simulink model "PD_LargeTimeCons"  (R2020b)
(part 4 of 4)

    td2*(td1*(0.00084023437500000005238864897449957*cos(t1)*cos(t5)*sin(t1) + 0.00042011718750000002619432448724979*cos(t1)^2*cos(t2)*cos(t3)*cos(t4)*sin(t5) - 0.00042011718750000002619432448724979*cos(t2)*cos(t3)*cos(t4)*sin(t1)^2*sin(t5) - 0.00042011718750000002619432448724979*cos(t1)^2*cos(t2)*sin(t3)*sin(t4)*sin(t5) - 0.00042011718750000002619432448724979*cos(t1)^2*cos(t3)*sin(t2)*sin(t4)*sin(t5) - 0.00042011718750000002619432448724979*cos(t1)^2*cos(t4)*sin(t2)*sin(t3)*sin(t5) + 0.00042011718750000002619432448724979*cos(t2)*sin(t1)^2*sin(t3)*sin(t4)*sin(t5) + 0.00042011718750000002619432448724979*cos(t3)*sin(t1)^2*sin(t2)*sin(t4)*sin(t5) + 0.00042011718750000002619432448724979*cos(t4)*sin(t1)^2*sin(t2)*sin(t3)*sin(t5)) + td6*(0.5*(0.00084023437500000005238864897449957*cos(t1)*cos(t2)*cos(t3)*sin(t4)*sin(t5) + 0.00084023437500000005238864897449957*cos(t1)*cos(t2)*cos(t4)*sin(t3)*sin(t5) + 0.00084023437500000005238864897449957*cos(t1)*cos(t3)*cos(t4)*sin(t2)*sin(t5) - 0.00084023437500000005238864897449957*cos(t1)*sin(t2)*sin(t3)*sin(t4)*sin(t5))*(cos(t1)*cos(t2)*sin(t3)*sin(t4)*sin(t5) - 1.0*cos(t1)*cos(t2)*cos(t3)*cos(t4)*sin(t5) - 1.0*cos(t5)*sin(t1) + cos(t1)*cos(t3)*sin(t2)*sin(t4)*sin(t5) + cos(t1)*cos(t4)*sin(t2)*sin(t3)*sin(t5)) + 0.5*(cos(t1)*cos(t2)*cos(t3)*sin(t4)*sin(t5) + cos(t1)*cos(t2)*cos(t4)*sin(t3)*sin(t5) + cos(t1)*cos(t3)*cos(t4)*sin(t2)*sin(t5) - 1.0*cos(t1)*sin(t2)*sin(t3)*sin(t4)*sin(t5))*(0.00084023437500000005238864897449957*cos(t1)*cos(t2)*sin(t3)*sin(t4)*sin(t5) - 0.00084023437500000005238864897449957*cos(t1)*cos(t2)*cos(t3)*cos(t4)*sin(t5) - 0.00084023437500000005238864897449957*cos(t5)*sin(t1) + 0.00084023437500000005238864897449957*cos(t1)*cos(t3)*sin(t2)*sin(t4)*sin(t5) + 0.00084023437500000005238864897449957*cos(t1)*cos(t4)*sin(t2)*sin(t3)*sin(t5)) + 0.5*(0.0016804687500000001047772979489991*cos(t2)*cos(t3)*sin(t1)*sin(t4)*sin(t5) + 0.0016804687500000001047772979489991*cos(t2)*cos(t4)*sin(t1)*sin(t3)*sin(t5) + 0.0016804687500000001047772979489991*cos(t3)*cos(t4)*sin(t1)*sin(t2)*sin(t5) - 0.0016804687500000001047772979489991*sin(t1)*sin(t2)*sin(t3)*sin(t4)*sin(t5))*(cos(t1)*cos(t5) - 1.0*cos(t2)*cos(t3)*cos(t4)*sin(t1)*sin(t5) + cos(t2)*sin(t1)*sin(t3)*sin(t4)*sin(t5) + cos(t3)*sin(t1)*sin(t2)*sin(t4)*sin(t5) + cos(t4)*sin(t1)*sin(t2)*sin(t3)*sin(t5)) + 0.5*(cos(t2)*cos(t3)*sin(t1)*sin(t4)*sin(t5) + cos(t2)*cos(t4)*sin(t1)*sin(t3)*sin(t5) + cos(t3)*cos(t4)*sin(t1)*sin(t2)*sin(t5) - 1.0*sin(t1)*sin(t2)*sin(t3)*sin(t4)*sin(t5))*(0.0016804687500000001047772979489991*cos(t1)*cos(t5) - 0.0016804687500000001047772979489991*cos(t2)*cos(t3)*cos(t4)*sin(t1)*sin(t5) + 0.0016804687500000001047772979489991*cos(t2)*sin(t1)*sin(t3)*sin(t4)*sin(t5) + 0.0016804687500000001047772979489991*cos(t3)*sin(t1)*sin(t2)*sin(t4)*sin(t5) + 0.0016804687500000001047772979489991*cos(t4)*sin(t1)*sin(t2)*sin(t3)*sin(t5))) - 1.0*td5*(0.00063017578125000003929148673087468*cos(2.0*t2)*cos(2.0*t3)*cos(2.0*t4)*sin(t5) - 0.00042011718750000002619432448724979*cos(t1)^2*sin(t5) - 0.00042011718750000002619432448724979*sin(t5) - 0.00063017578125000003929148673087468*cos(2.0*t2)*sin(2.0*t3)*sin(2.0*t4)*sin(t5) - 0.00063017578125000003929148673087468*cos(2.0*t3)*sin(2.0*t2)*sin(2.0*t4)*sin(t5) - 0.00063017578125000003929148673087468*cos(2.0*t4)*sin(2.0*t2)*sin(2.0*t3)*sin(t5) - 0.00021005859375000001309716224362489*cos(2.0*t1)*cos(2.0*t2)*cos(2.0*t3)*cos(2.0*t4)*sin(t5) + 0.00021005859375000001309716224362489*cos(2.0*t1)*cos(2.0*t2)*sin(2.0*t3)*sin(2.0*t4)*sin(t5) + 0.00021005859375000001309716224362489*cos(2.0*t1)*cos(2.0*t3)*sin(2.0*t2)*sin(2.0*t4)*sin(t5) + 0.00021005859375000001309716224362489*cos(2.0*t1)*cos(2.0*t4)*sin(2.0*t2)*sin(2.0*t3)*sin(t5) - 0.00021005859375000001309716224362489*sin(2.0*t1)*cos(t2)*cos(t3)*cos(t4)*cos(t5) + 0.00021005859375000001309716224362489*sin(2.0*t1)*cos(t2)*cos(t5)*sin(t3)*sin(t4) + 0.00021005859375000001309716224362489*sin(2.0*t1)*cos(t3)*cos(t5)*sin(t2)*sin(t4) + 0.00021005859375000001309716224362489*sin(2.0*t1)*cos(t4)*cos(t5)*sin(t2)*sin(t3) - 0.00042011718750000002619432448724979*cos(t1)*cos(t2)*cos(t3)*cos(t4)*cos(t5)*sin(t1) + 0.00042011718750000002619432448724979*cos(t1)*cos(t2)*cos(t5)*sin(t1)*sin(t3)*sin(t4) + 0.00042011718750000002619432448724979*cos(t1)*cos(t3)*cos(t5)*sin(t1)*sin(t2)*sin(t4) + 0.00042011718750000002619432448724979*cos(t1)*cos(t4)*cos(t5)*sin(t1)*sin(t2)*sin(t3))) + td3*(td1*(0.00084023437500000005238864897449957*cos(t1)*cos(t5)*sin(t1) + 0.00042011718750000002619432448724979*cos(t1)^2*cos(t2)*cos(t3)*cos(t4)*sin(t5) - 0.00042011718750000002619432448724979*cos(t2)*cos(t3)*cos(t4)*sin(t1)^2*sin(t5) - 0.00042011718750000002619432448724979*cos(t1)^2*cos(t2)*sin(t3)*sin(t4)*sin(t5) - 0.00042011718750000002619432448724979*cos(t1)^2*cos(t3)*sin(t2)*sin(t4)*sin(t5) - 0.00042011718750000002619432448724979*cos(t1)^2*cos(t4)*sin(t2)*sin(t3)*sin(t5) + 0.00042011718750000002619432448724979*cos(t2)*sin(t1)^2*sin(t3)*sin(t4)*sin(t5) + 0.00042011718750000002619432448724979*cos(t3)*sin(t1)^2*sin(t2)*sin(t4)*sin(t5) + 0.00042011718750000002619432448724979*cos(t4)*sin(t1)^2*sin(t2)*sin(t3)*sin(t5)) + td6*(0.5*(0.00084023437500000005238864897449957*cos(t1)*cos(t2)*cos(t3)*sin(t4)*sin(t5) + 0.00084023437500000005238864897449957*cos(t1)*cos(t2)*cos(t4)*sin(t3)*sin(t5) + 0.00084023437500000005238864897449957*cos(t1)*cos(t3)*cos(t4)*sin(t2)*sin(t5) - 0.00084023437500000005238864897449957*cos(t1)*sin(t2)*sin(t3)*sin(t4)*sin(t5))*(cos(t1)*cos(t2)*sin(t3)*sin(t4)*sin(t5) - 1.0*cos(t1)*cos(t2)*cos(t3)*cos(t4)*sin(t5) - 1.0*cos(t5)*sin(t1) + cos(t1)*cos(t3)*sin(t2)*sin(t4)*sin(t5) + cos(t1)*cos(t4)*sin(t2)*sin(t3)*sin(t5)) + 0.5*(cos(t1)*cos(t2)*cos(t3)*sin(t4)*sin(t5) + cos(t1)*cos(t2)*cos(t4)*sin(t3)*sin(t5) + cos(t1)*cos(t3)*cos(t4)*sin(t2)*sin(t5) - 1.0*cos(t1)*sin(t2)*sin(t3)*sin(t4)*sin(t5))*(0.00084023437500000005238864897449957*cos(t1)*cos(t2)*sin(t3)*sin(t4)*sin(t5) - 0.00084023437500000005238864897449957*cos(t1)*cos(t2)*cos(t3)*cos(t4)*sin(t5) - 0.00084023437500000005238864897449957*cos(t5)*sin(t1) + 0.00084023437500000005238864897449957*cos(t1)*cos(t3)*sin(t2)*sin(t4)*sin(t5) + 0.00084023437500000005238864897449957*cos(t1)*cos(t4)*sin(t2)*sin(t3)*sin(t5)) + 0.5*(0.0016804687500000001047772979489991*cos(t2)*cos(t3)*sin(t1)*sin(t4)*sin(t5) + 0.0016804687500000001047772979489991*cos(t2)*cos(t4)*sin(t1)*sin(t3)*sin(t5) + 0.0016804687500000001047772979489991*cos(t3)*cos(t4)*sin(t1)*sin(t2)*sin(t5) - 0.0016804687500000001047772979489991*sin(t1)*sin(t2)*sin(t3)*sin(t4)*sin(t5))*(cos(t1)*cos(t5) - 1.0*cos(t2)*cos(t3)*cos(t4)*sin(t1)*sin(t5) + cos(t2)*sin(t1)*sin(t3)*sin(t4)*sin(t5) + cos(t3)*sin(t1)*sin(t2)*sin(t4)*sin(t5) + cos(t4)*sin(t1)*sin(t2)*sin(t3)*sin(t5)) + 0.5*(cos(t2)*cos(t3)*sin(t1)*sin(t4)*sin(t5) + cos(t2)*cos(t4)*sin(t1)*sin(t3)*sin(t5) + cos(t3)*cos(t4)*sin(t1)*sin(t2)*sin(t5) - 1.0*sin(t1)*sin(t2)*sin(t3)*sin(t4)*sin(t5))*(0.0016804687500000001047772979489991*cos(t1)*cos(t5) - 0.0016804687500000001047772979489991*cos(t2)*cos(t3)*cos(t4)*sin(t1)*sin(t5) + 0.0016804687500000001047772979489991*cos(t2)*sin(t1)*sin(t3)*sin(t4)*sin(t5) + 0.0016804687500000001047772979489991*cos(t3)*sin(t1)*sin(t2)*sin(t4)*sin(t5) + 0.0016804687500000001047772979489991*cos(t4)*sin(t1)*sin(t2)*sin(t3)*sin(t5))) - 1.0*td5*(0.00063017578125000003929148673087468*cos(2.0*t2)*cos(2.0*t3)*cos(2.0*t4)*sin(t5) - 0.00042011718750000002619432448724979*cos(t1)^2*sin(t5) - 0.00042011718750000002619432448724979*sin(t5) - 0.00063017578125000003929148673087468*cos(2.0*t2)*sin(2.0*t3)*sin(2.0*t4)*sin(t5) - 0.00063017578125000003929148673087468*cos(2.0*t3)*sin(2.0*t2)*sin(2.0*t4)*sin(t5) - 0.00063017578125000003929148673087468*cos(2.0*t4)*sin(2.0*t2)*sin(2.0*t3)*sin(t5) - 0.00021005859375000001309716224362489*cos(2.0*t1)*cos(2.0*t2)*cos(2.0*t3)*cos(2.0*t4)*sin(t5) + 0.00021005859375000001309716224362489*cos(2.0*t1)*cos(2.0*t2)*sin(2.0*t3)*sin(2.0*t4)*sin(t5) + 0.00021005859375000001309716224362489*cos(2.0*t1)*cos(2.0*t3)*sin(2.0*t2)*sin(2.0*t4)*sin(t5) + 0.00021005859375000001309716224362489*cos(2.0*t1)*cos(2.0*t4)*sin(2.0*t2)*sin(2.0*t3)*sin(t5) - 0.00021005859375000001309716224362489*sin(2.0*t1)*cos(t2)*cos(t3)*cos(t4)*cos(t5) + 0.00021005859375000001309716224362489*sin(2.0*t1)*cos(t2)*cos(t5)*sin(t3)*sin(t4) + 0.00021005859375000001309716224362489*sin(2.0*t1)*cos(t3)*cos(t5)*sin(t2)*sin(t4) + 0.00021005859375000001309716224362489*sin(2.0*t1)*cos(t4)*cos(t5)*sin(t2)*sin(t3) - 0.00042011718750000002619432448724979*cos(t1)*cos(t2)*cos(t3)*cos(t4)*cos(t5)*sin(t1) + 0.00042011718750000002619432448724979*cos(t1)*cos(t2)*cos(t5)*sin(t1)*sin(t3)*sin(t4) + 0.00042011718750000002619432448724979*cos(t1)*cos(t3)*cos(t5)*sin(t1)*sin(t2)*sin(t4) + 0.00042011718750000002619432448724979*cos(t1)*cos(t4)*cos(t5)*sin(t1)*sin(t2)*sin(t3))) + td4*(td1*(0.00084023437500000005238864897449957*cos(t1)*cos(t5)*sin(t1) + 0.00042011718750000002619432448724979*cos(t1)^2*cos(t2)*cos(t3)*cos(t4)*sin(t5) - 0.00042011718750000002619432448724979*cos(t2)*cos(t3)*cos(t4)*sin(t1)^2*sin(t5) - 0.00042011718750000002619432448724979*cos(t1)^2*cos(t2)*sin(t3)*sin(t4)*sin(t5) - 0.00042011718750000002619432448724979*cos(t1)^2*cos(t3)*sin(t2)*sin(t4)*sin(t5) - 0.00042011718750000002619432448724979*cos(t1)^2*cos(t4)*sin(t2)*sin(t3)*sin(t5) + 0.00042011718750000002619432448724979*cos(t2)*sin(t1)^2*sin(t3)*sin(t4)*sin(t5) + 0.00042011718750000002619432448724979*cos(t3)*sin(t1)^2*sin(t2)*sin(t4)*sin(t5) + 0.00042011718750000002619432448724979*cos(t4)*sin(t1)^2*sin(t2)*sin(t3)*sin(t5)) + td6*(0.5*(0.00084023437500000005238864897449957*cos(t1)*cos(t2)*cos(t3)*sin(t4)*sin(t5) + 0.00084023437500000005238864897449957*cos(t1)*cos(t2)*cos(t4)*sin(t3)*sin(t5) + 0.00084023437500000005238864897449957*cos(t1)*cos(t3)*cos(t4)*sin(t2)*sin(t5) - 0.00084023437500000005238864897449957*cos(t1)*sin(t2)*sin(t3)*sin(t4)*sin(t5))*(cos(t1)*cos(t2)*sin(t3)*sin(t4)*sin(t5) - 1.0*cos(t1)*cos(t2)*cos(t3)*cos(t4)*sin(t5) - 1.0*cos(t5)*sin(t1) + cos(t1)*cos(t3)*sin(t2)*sin(t4)*sin(t5) + cos(t1)*cos(t4)*sin(t2)*sin(t3)*sin(t5)) + 0.5*(cos(t1)*cos(t2)*cos(t3)*sin(t4)*sin(t5) + cos(t1)*cos(t2)*cos(t4)*sin(t3)*sin(t5) + cos(t1)*cos(t3)*cos(t4)*sin(t2)*sin(t5) - 1.0*cos(t1)*sin(t2)*sin(t3)*sin(t4)*sin(t5))*(0.00084023437500000005238864897449957*cos(t1)*cos(t2)*sin(t3)*sin(t4)*sin(t5) - 0.00084023437500000005238864897449957*cos(t1)*cos(t2)*cos(t3)*cos(t4)*sin(t5) - 0.00084023437500000005238864897449957*cos(t5)*sin(t1) + 0.00084023437500000005238864897449957*cos(t1)*cos(t3)*sin(t2)*sin(t4)*sin(t5) + 0.00084023437500000005238864897449957*cos(t1)*cos(t4)*sin(t2)*sin(t3)*sin(t5)) + 0.5*(0.0016804687500000001047772979489991*cos(t2)*cos(t3)*sin(t1)*sin(t4)*sin(t5) + 0.0016804687500000001047772979489991*cos(t2)*cos(t4)*sin(t1)*sin(t3)*sin(t5) + 0.0016804687500000001047772979489991*cos(t3)*cos(t4)*sin(t1)*sin(t2)*sin(t5) - 0.0016804687500000001047772979489991*sin(t1)*sin(t2)*sin(t3)*sin(t4)*sin(t5))*(cos(t1)*cos(t5) - 1.0*cos(t2)*cos(t3)*cos(t4)*sin(t1)*sin(t5) + cos(t2)*sin(t1)*sin(t3)*sin(t4)*sin(t5) + cos(t3)*sin(t1)*sin(t2)*sin(t4)*sin(t5) + cos(t4)*sin(t1)*sin(t2)*sin(t3)*sin(t5)) + 0.5*(cos(t2)*cos(t3)*sin(t1)*sin(t4)*sin(t5) + cos(t2)*cos(t4)*sin(t1)*sin(t3)*sin(t5) + cos(t3)*cos(t4)*sin(t1)*sin(t2)*sin(t5) - 1.0*sin(t1)*sin(t2)*sin(t3)*sin(t4)*sin(t5))*(0.0016804687500000001047772979489991*cos(t1)*cos(t5) - 0.0016804687500000001047772979489991*cos(t2)*cos(t3)*cos(t4)*sin(t1)*sin(t5) + 0.0016804687500000001047772979489991*cos(t2)*sin(t1)*sin(t3)*sin(t4)*sin(t5) + 0.0016804687500000001047772979489991*cos(t3)*sin(t1)*sin(t2)*sin(t4)*sin(t5) + 0.0016804687500000001047772979489991*cos(t4)*sin(t1)*sin(t2)*sin(t3)*sin(t5))) - 1.0*td5*(0.00063017578125000003929148673087468*cos(2.0*t2)*cos(2.0*t3)*cos(2.0*t4)*sin(t5) - 0.00042011718750000002619432448724979*cos(t1)^2*sin(t5) - 0.00042011718750000002619432448724979*sin(t5) - 0.00063017578125000003929148673087468*cos(2.0*t2)*sin(2.0*t3)*sin(2.0*t4)*sin(t5) - 0.00063017578125000003929148673087468*cos(2.0*t3)*sin(2.0*t2)*sin(2.0*t4)*sin(t5) - 0.00063017578125000003929148673087468*cos(2.0*t4)*sin(2.0*t2)*sin(2.0*t3)*sin(t5) - 0.00021005859375000001309716224362489*cos(2.0*t1)*cos(2.0*t2)*cos(2.0*t3)*cos(2.0*t4)*sin(t5) + 0.00021005859375000001309716224362489*cos(2.0*t1)*cos(2.0*t2)*sin(2.0*t3)*sin(2.0*t4)*sin(t5) + 0.00021005859375000001309716224362489*cos(2.0*t1)*cos(2.0*t3)*sin(2.0*t2)*sin(2.0*t4)*sin(t5) + 0.00021005859375000001309716224362489*cos(2.0*t1)*cos(2.0*t4)*sin(2.0*t2)*sin(2.0*t3)*sin(t5) - 0.00021005859375000001309716224362489*sin(2.0*t1)*cos(t2)*cos(t3)*cos(t4)*cos(t5) + 0.00021005859375000001309716224362489*sin(2.0*t1)*cos(t2)*cos(t5)*sin(t3)*sin(t4) + 0.00021005859375000001309716224362489*sin(2.0*t1)*cos(t3)*cos(t5)*sin(t2)*sin(t4) + 0.00021005859375000001309716224362489*sin(2.0*t1)*cos(t4)*cos(t5)*sin(t2)*sin(t3) - 0.00042011718750000002619432448724979*cos(t1)*cos(t2)*cos(t3)*cos(t4)*cos(t5)*sin(t1) + 0.00042011718750000002619432448724979*cos(t1)*cos(t2)*cos(t5)*sin(t1)*sin(t3)*sin(t4) + 0.00042011718750000002619432448724979*cos(t1)*cos(t3)*cos(t5)*sin(t1)*sin(t2)*sin(t4) + 0.00042011718750000002619432448724979*cos(t1)*cos(t4)*cos(t5)*sin(t1)*sin(t2)*sin(t3))) - td1*(td6*(0.5*(0.00084023437500000005238864897449957*cos(t1)*cos(t5) - 0.00084023437500000005238864897449957*cos(t2)*cos(t3)*cos(t4)*sin(t1)*sin(t5) + 0.00084023437500000005238864897449957*cos(t2)*sin(t1)*sin(t3)*sin(t4)*sin(t5) + 0.00084023437500000005238864897449957*cos(t3)*sin(t1)*sin(t2)*sin(t4)*sin(t5) + 0.00084023437500000005238864897449957*cos(t4)*sin(t1)*sin(t2)*sin(t3)*sin(t5))*(cos(t1)*cos(t2)*sin(t3)*sin(t4)*sin(t5) - 1.0*cos(t1)*cos(t2)*cos(t3)*cos(t4)*sin(t5) - 1.0*cos(t5)*sin(t1) + cos(t1)*cos(t3)*sin(t2)*sin(t4)*sin(t5) + cos(t1)*cos(t4)*sin(t2)*sin(t3)*sin(t5)) - 0.5*(0.0016804687500000001047772979489991*cos(t1)*cos(t5) - 0.0016804687500000001047772979489991*cos(t2)*cos(t3)*cos(t4)*sin(t1)*sin(t5) + 0.0016804687500000001047772979489991*cos(t2)*sin(t1)*sin(t3)*sin(t4)*sin(t5) + 0.0016804687500000001047772979489991*cos(t3)*sin(t1)*sin(t2)*sin(t4)*sin(t5) + 0.0016804687500000001047772979489991*cos(t4)*sin(t1)*sin(t2)*sin(t3)*sin(t5))*(cos(t1)*cos(t2)*sin(t3)*sin(t4)*sin(t5) - 1.0*cos(t1)*cos(t2)*cos(t3)*cos(t4)*sin(t5) - 1.0*cos(t5)*sin(t1) + cos(t1)*cos(t3)*sin(t2)*sin(t4)*sin(t5) + cos(t1)*cos(t4)*sin(t2)*sin(t3)*sin(t5)) + 0.5*(0.00084023437500000005238864897449957*cos(t1)*cos(t2)*sin(t3)*sin(t4)*sin(t5) - 0.00084023437500000005238864897449957*cos(t1)*cos(t2)*cos(t3)*cos(t4)*sin(t5) - 0.00084023437500000005238864897449957*cos(t5)*sin(t1) + 0.00084023437500000005238864897449957*cos(t1)*cos(t3)*sin(t2)*sin(t4)*sin(t5) + 0.00084023437500000005238864897449957*cos(t1)*cos(t4)*sin(t2)*sin(t3)*sin(t5))*(cos(t1)*cos(t5) - 1.0*cos(t2)*cos(t3)*cos(t4)*sin(t1)*sin(t5) + cos(t2)*sin(t1)*sin(t3)*sin(t4)*sin(t5) + cos(t3)*sin(t1)*sin(t2)*sin(t4)*sin(t5) + cos(t4)*sin(t1)*sin(t2)*sin(t3)*sin(t5)) - 0.5*(0.0016804687500000001047772979489991*cos(t1)*cos(t2)*sin(t3)*sin(t4)*sin(t5) - 0.0016804687500000001047772979489991*cos(t1)*cos(t2)*cos(t3)*cos(t4)*sin(t5) - 0.0016804687500000001047772979489991*cos(t5)*sin(t1) + 0.0016804687500000001047772979489991*cos(t1)*cos(t3)*sin(t2)*sin(t4)*sin(t5) + 0.0016804687500000001047772979489991*cos(t1)*cos(t4)*sin(t2)*sin(t3)*sin(t5))*(cos(t1)*cos(t5) - 1.0*cos(t2)*cos(t3)*cos(t4)*sin(t1)*sin(t5) + cos(t2)*sin(t1)*sin(t3)*sin(t4)*sin(t5) + cos(t3)*sin(t1)*sin(t2)*sin(t4)*sin(t5) + cos(t4)*sin(t1)*sin(t2)*sin(t3)*sin(t5))) + 1.0*td2*(0.00084023437500000005238864897449957*cos(t1)*cos(t5)*sin(t1) + 0.00042011718750000002619432448724979*cos(t1)^2*cos(t2)*cos(t3)*cos(t4)*sin(t5) - 0.00042011718750000002619432448724979*cos(t2)*cos(t3)*cos(t4)*sin(t1)^2*sin(t5) - 0.00042011718750000002619432448724979*cos(t1)^2*cos(t2)*sin(t3)*sin(t4)*sin(t5) - 0.00042011718750000002619432448724979*cos(t1)^2*cos(t3)*sin(t2)*sin(t4)*sin(t5) - 0.00042011718750000002619432448724979*cos(t1)^2*cos(t4)*sin(t2)*sin(t3)*sin(t5) + 0.00042011718750000002619432448724979*cos(t2)*sin(t1)^2*sin(t3)*sin(t4)*sin(t5) + 0.00042011718750000002619432448724979*cos(t3)*sin(t1)^2*sin(t2)*sin(t4)*sin(t5) + 0.00042011718750000002619432448724979*cos(t4)*sin(t1)^2*sin(t2)*sin(t3)*sin(t5)) + 1.0*td3*(0.00084023437500000005238864897449957*cos(t1)*cos(t5)*sin(t1) + 0.00042011718750000002619432448724979*cos(t1)^2*cos(t2)*cos(t3)*cos(t4)*sin(t5) - 0.00042011718750000002619432448724979*cos(t2)*cos(t3)*cos(t4)*sin(t1)^2*sin(t5) - 0.00042011718750000002619432448724979*cos(t1)^2*cos(t2)*sin(t3)*sin(t4)*sin(t5) - 0.00042011718750000002619432448724979*cos(t1)^2*cos(t3)*sin(t2)*sin(t4)*sin(t5) - 0.00042011718750000002619432448724979*cos(t1)^2*cos(t4)*sin(t2)*sin(t3)*sin(t5) + 0.00042011718750000002619432448724979*cos(t2)*sin(t1)^2*sin(t3)*sin(t4)*sin(t5) + 0.00042011718750000002619432448724979*cos(t3)*sin(t1)^2*sin(t2)*sin(t4)*sin(t5) + 0.00042011718750000002619432448724979*cos(t4)*sin(t1)^2*sin(t2)*sin(t3)*sin(t5)) + 1.0*td4*(0.00084023437500000005238864897449957*cos(t1)*cos(t5)*sin(t1) + 0.00042011718750000002619432448724979*cos(t1)^2*cos(t2)*cos(t3)*cos(t4)*sin(t5) - 0.00042011718750000002619432448724979*cos(t2)*cos(t3)*cos(t4)*sin(t1)^2*sin(t5) - 0.00042011718750000002619432448724979*cos(t1)^2*cos(t2)*sin(t3)*sin(t4)*sin(t5) - 0.00042011718750000002619432448724979*cos(t1)^2*cos(t3)*sin(t2)*sin(t4)*sin(t5) - 0.00042011718750000002619432448724979*cos(t1)^2*cos(t4)*sin(t2)*sin(t3)*sin(t5) + 0.00042011718750000002619432448724979*cos(t2)*sin(t1)^2*sin(t3)*sin(t4)*sin(t5) + 0.00042011718750000002619432448724979*cos(t3)*sin(t1)^2*sin(t2)*sin(t4)*sin(t5) + 0.00042011718750000002619432448724979*cos(t4)*sin(t1)^2*sin(t2)*sin(t3)*sin(t5)) + td5*(0.00021005859375000001309716224362489*cos(2.0*t2)*cos(2.0*t3)*sin(2.0*t1)*sin(2.0*t4)*sin(t5) + 0.00021005859375000001309716224362489*cos(2.0*t2)*cos(2.0*t4)*sin(2.0*t1)*sin(2.0*t3)*sin(t5) + 0.00021005859375000001309716224362489*cos(2.0*t3)*cos(2.0*t4)*sin(2.0*t1)*sin(2.0*t2)*sin(t5) - 0.00042011718750000002619432448724979*cos(2.0*t1)*cos(t2)*cos(t3)*cos(t5)*sin(t4) - 0.00042011718750000002619432448724979*cos(2.0*t1)*cos(t2)*cos(t4)*cos(t5)*sin(t3) - 0.00042011718750000002619432448724979*cos(2.0*t1)*cos(t3)*cos(t4)*cos(t5)*sin(t2) - 0.00021005859375000001309716224362489*sin(2.0*t1)*sin(2.0*t2)*sin(2.0*t3)*sin(2.0*t4)*sin(t5) + 0.00042011718750000002619432448724979*cos(2.0*t1)*cos(t5)*sin(t2)*sin(t3)*sin(t4))) - td6*(1.0*td5*(0.5*(0.0016804687500000001047772979489991*cos(t1)*cos(t5) - 0.0016804687500000001047772979489991*cos(t2)*cos(t3)*cos(t4)*sin(t1)*sin(t5) + 0.0016804687500000001047772979489991*cos(t2)*sin(t1)*sin(t3)*sin(t4)*sin(t5) + 0.0016804687500000001047772979489991*cos(t3)*sin(t1)*sin(t2)*sin(t4)*sin(t5) + 0.0016804687500000001047772979489991*cos(t4)*sin(t1)*sin(t2)*sin(t3)*sin(t5))*(cos(t2)*cos(t5)*sin(t1)*sin(t3)*sin(t4) - 1.0*cos(t2)*cos(t3)*cos(t4)*cos(t5)*sin(t1) - 1.0*cos(t1)*sin(t5) + cos(t3)*cos(t5)*sin(t1)*sin(t2)*sin(t4) + cos(t4)*cos(t5)*sin(t1)*sin(t2)*sin(t3)) + 0.5*(sin(t1)*sin(t5) - 1.0*cos(t1)*cos(t2)*cos(t3)*cos(t4)*cos(t5) + cos(t1)*cos(t2)*cos(t5)*sin(t3)*sin(t4) + cos(t1)*cos(t3)*cos(t5)*sin(t2)*sin(t4) + cos(t1)*cos(t4)*cos(t5)*sin(t2)*sin(t3))*(0.00084023437500000005238864897449957*cos(t1)*cos(t2)*sin(t3)*sin(t4)*sin(t5) - 0.00084023437500000005238864897449957*cos(t1)*cos(t2)*cos(t3)*cos(t4)*sin(t5) - 0.00084023437500000005238864897449957*cos(t5)*sin(t1) + 0.00084023437500000005238864897449957*cos(t1)*cos(t3)*sin(t2)*sin(t4)*sin(t5) + 0.00084023437500000005238864897449957*cos(t1)*cos(t4)*sin(t2)*sin(t3)*sin(t5)) + 0.5*(0.00084023437500000005238864897449957*sin(t1)*sin(t5) - 0.00084023437500000005238864897449957*cos(t1)*cos(t2)*cos(t3)*cos(t4)*cos(t5) + 0.00084023437500000005238864897449957*cos(t1)*cos(t2)*cos(t5)*sin(t3)*sin(t4) + 0.00084023437500000005238864897449957*cos(t1)*cos(t3)*cos(t5)*sin(t2)*sin(t4) + 0.00084023437500000005238864897449957*cos(t1)*cos(t4)*cos(t5)*sin(t2)*sin(t3))*(cos(t1)*cos(t2)*sin(t3)*sin(t4)*sin(t5) - 1.0*cos(t1)*cos(t2)*cos(t3)*cos(t4)*sin(t5) - 1.0*cos(t5)*sin(t1) + cos(t1)*cos(t3)*sin(t2)*sin(t4)*sin(t5) + cos(t1)*cos(t4)*sin(t2)*sin(t3)*sin(t5)) + 0.5*(0.0016804687500000001047772979489991*cos(t2)*cos(t5)*sin(t1)*sin(t3)*sin(t4) - 0.0016804687500000001047772979489991*cos(t2)*cos(t3)*cos(t4)*cos(t5)*sin(t1) - 0.0016804687500000001047772979489991*cos(t1)*sin(t5) + 0.0016804687500000001047772979489991*cos(t3)*cos(t5)*sin(t1)*sin(t2)*sin(t4) + 0.0016804687500000001047772979489991*cos(t4)*cos(t5)*sin(t1)*sin(t2)*sin(t3))*(cos(t1)*cos(t5) - 1.0*cos(t2)*cos(t3)*cos(t4)*sin(t1)*sin(t5) + cos(t2)*sin(t1)*sin(t3)*sin(t4)*sin(t5) + cos(t3)*sin(t1)*sin(t2)*sin(t4)*sin(t5) + cos(t4)*sin(t1)*sin(t2)*sin(t3)*sin(t5))) - 1.0*td1*(0.5*(0.00084023437500000005238864897449957*cos(t1)*cos(t5) - 0.00084023437500000005238864897449957*cos(t2)*cos(t3)*cos(t4)*sin(t1)*sin(t5) + 0.00084023437500000005238864897449957*cos(t2)*sin(t1)*sin(t3)*sin(t4)*sin(t5) + 0.00084023437500000005238864897449957*cos(t3)*sin(t1)*sin(t2)*sin(t4)*sin(t5) + 0.00084023437500000005238864897449957*cos(t4)*sin(t1)*sin(t2)*sin(t3)*sin(t5))*(cos(t1)*cos(t2)*sin(t3)*sin(t4)*sin(t5) - 1.0*cos(t1)*cos(t2)*cos(t3)*cos(t4)*sin(t5) - 1.0*cos(t5)*sin(t1) + cos(t1)*cos(t3)*sin(t2)*sin(t4)*sin(t5) + cos(t1)*cos(t4)*sin(t2)*sin(t3)*sin(t5)) - 0.5*(0.0016804687500000001047772979489991*cos(t1)*cos(t5) - 0.0016804687500000001047772979489991*cos(t2)*cos(t3)*cos(t4)*sin(t1)*sin(t5) + 0.0016804687500000001047772979489991*cos(t2)*sin(t1)*sin(t3)*sin(t4)*sin(t5) + 0.0016804687500000001047772979489991*cos(t3)*sin(t1)*sin(t2)*sin(t4)*sin(t5) + 0.0016804687500000001047772979489991*cos(t4)*sin(t1)*sin(t2)*sin(t3)*sin(t5))*(cos(t1)*cos(t2)*sin(t3)*sin(t4)*sin(t5) - 1.0*cos(t1)*cos(t2)*cos(t3)*cos(t4)*sin(t5) - 1.0*cos(t5)*sin(t1) + cos(t1)*cos(t3)*sin(t2)*sin(t4)*sin(t5) + cos(t1)*cos(t4)*sin(t2)*sin(t3)*sin(t5)) + 0.5*(0.00084023437500000005238864897449957*cos(t1)*cos(t2)*sin(t3)*sin(t4)*sin(t5) - 0.00084023437500000005238864897449957*cos(t1)*cos(t2)*cos(t3)*cos(t4)*sin(t5) - 0.00084023437500000005238864897449957*cos(t5)*sin(t1) + 0.00084023437500000005238864897449957*cos(t1)*cos(t3)*sin(t2)*sin(t4)*sin(t5) + 0.00084023437500000005238864897449957*cos(t1)*cos(t4)*sin(t2)*sin(t3)*sin(t5))*(cos(t1)*cos(t5) - 1.0*cos(t2)*cos(t3)*cos(t4)*sin(t1)*sin(t5) + cos(t2)*sin(t1)*sin(t3)*sin(t4)*sin(t5) + cos(t3)*sin(t1)*sin(t2)*sin(t4)*sin(t5) + cos(t4)*sin(t1)*sin(t2)*sin(t3)*sin(t5)) - 0.5*(0.0016804687500000001047772979489991*cos(t1)*cos(t2)*sin(t3)*sin(t4)*sin(t5) - 0.0016804687500000001047772979489991*cos(t1)*cos(t2)*cos(t3)*cos(t4)*sin(t5) - 0.0016804687500000001047772979489991*cos(t5)*sin(t1) + 0.0016804687500000001047772979489991*cos(t1)*cos(t3)*sin(t2)*sin(t4)*sin(t5) + 0.0016804687500000001047772979489991*cos(t1)*cos(t4)*sin(t2)*sin(t3)*sin(t5))*(cos(t1)*cos(t5) - 1.0*cos(t2)*cos(t3)*cos(t4)*sin(t1)*sin(t5) + cos(t2)*sin(t1)*sin(t3)*sin(t4)*sin(t5) + cos(t3)*sin(t1)*sin(t2)*sin(t4)*sin(t5) + cos(t4)*sin(t1)*sin(t2)*sin(t3)*sin(t5))) + 1.0*td2*(0.5*(0.00084023437500000005238864897449957*cos(t1)*cos(t2)*cos(t3)*sin(t4)*sin(t5) + 0.00084023437500000005238864897449957*cos(t1)*cos(t2)*cos(t4)*sin(t3)*sin(t5) + 0.00084023437500000005238864897449957*cos(t1)*cos(t3)*cos(t4)*sin(t2)*sin(t5) - 0.00084023437500000005238864897449957*cos(t1)*sin(t2)*sin(t3)*sin(t4)*sin(t5))*(cos(t1)*cos(t2)*sin(t3)*sin(t4)*sin(t5) - 1.0*cos(t1)*cos(t2)*cos(t3)*cos(t4)*sin(t5) - 1.0*cos(t5)*sin(t1) + cos(t1)*cos(t3)*sin(t2)*sin(t4)*sin(t5) + cos(t1)*cos(t4)*sin(t2)*sin(t3)*sin(t5)) + 0.5*(cos(t1)*cos(t2)*cos(t3)*sin(t4)*sin(t5) + cos(t1)*cos(t2)*cos(t4)*sin(t3)*sin(t5) + cos(t1)*cos(t3)*cos(t4)*sin(t2)*sin(t5) - 1.0*cos(t1)*sin(t2)*sin(t3)*sin(t4)*sin(t5))*(0.00084023437500000005238864897449957*cos(t1)*cos(t2)*sin(t3)*sin(t4)*sin(t5) - 0.00084023437500000005238864897449957*cos(t1)*cos(t2)*cos(t3)*cos(t4)*sin(t5) - 0.00084023437500000005238864897449957*cos(t5)*sin(t1) + 0.00084023437500000005238864897449957*cos(t1)*cos(t3)*sin(t2)*sin(t4)*sin(t5) + 0.00084023437500000005238864897449957*cos(t1)*cos(t4)*sin(t2)*sin(t3)*sin(t5)) + 0.5*(0.0016804687500000001047772979489991*cos(t2)*cos(t3)*sin(t1)*sin(t4)*sin(t5) + 0.0016804687500000001047772979489991*cos(t2)*cos(t4)*sin(t1)*sin(t3)*sin(t5) + 0.0016804687500000001047772979489991*cos(t3)*cos(t4)*sin(t1)*sin(t2)*sin(t5) - 0.0016804687500000001047772979489991*sin(t1)*sin(t2)*sin(t3)*sin(t4)*sin(t5))*(cos(t1)*cos(t5) - 1.0*cos(t2)*cos(t3)*cos(t4)*sin(t1)*sin(t5) + cos(t2)*sin(t1)*sin(t3)*sin(t4)*sin(t5) + cos(t3)*sin(t1)*sin(t2)*sin(t4)*sin(t5) + cos(t4)*sin(t1)*sin(t2)*sin(t3)*sin(t5)) + 0.5*(cos(t2)*cos(t3)*sin(t1)*sin(t4)*sin(t5) + cos(t2)*cos(t4)*sin(t1)*sin(t3)*sin(t5) + cos(t3)*cos(t4)*sin(t1)*sin(t2)*sin(t5) - 1.0*sin(t1)*sin(t2)*sin(t3)*sin(t4)*sin(t5))*(0.0016804687500000001047772979489991*cos(t1)*cos(t5) - 0.0016804687500000001047772979489991*cos(t2)*cos(t3)*cos(t4)*sin(t1)*sin(t5) + 0.0016804687500000001047772979489991*cos(t2)*sin(t1)*sin(t3)*sin(t4)*sin(t5) + 0.0016804687500000001047772979489991*cos(t3)*sin(t1)*sin(t2)*sin(t4)*sin(t5) + 0.0016804687500000001047772979489991*cos(t4)*sin(t1)*sin(t2)*sin(t3)*sin(t5))) + 1.0*td3*(0.5*(0.00084023437500000005238864897449957*cos(t1)*cos(t2)*cos(t3)*sin(t4)*sin(t5) + 0.00084023437500000005238864897449957*cos(t1)*cos(t2)*cos(t4)*sin(t3)*sin(t5) + 0.00084023437500000005238864897449957*cos(t1)*cos(t3)*cos(t4)*sin(t2)*sin(t5) - 0.00084023437500000005238864897449957*cos(t1)*sin(t2)*sin(t3)*sin(t4)*sin(t5))*(cos(t1)*cos(t2)*sin(t3)*sin(t4)*sin(t5) - 1.0*cos(t1)*cos(t2)*cos(t3)*cos(t4)*sin(t5) - 1.0*cos(t5)*sin(t1) + cos(t1)*cos(t3)*sin(t2)*sin(t4)*sin(t5) + cos(t1)*cos(t4)*sin(t2)*sin(t3)*sin(t5)) + 0.5*(cos(t1)*cos(t2)*cos(t3)*sin(t4)*sin(t5) + cos(t1)*cos(t2)*cos(t4)*sin(t3)*sin(t5) + cos(t1)*cos(t3)*cos(t4)*sin(t2)*sin(t5) - 1.0*cos(t1)*sin(t2)*sin(t3)*sin(t4)*sin(t5))*(0.00084023437500000005238864897449957*cos(t1)*cos(t2)*sin(t3)*sin(t4)*sin(t5) - 0.00084023437500000005238864897449957*cos(t1)*cos(t2)*cos(t3)*cos(t4)*sin(t5) - 0.00084023437500000005238864897449957*cos(t5)*sin(t1) + 0.00084023437500000005238864897449957*cos(t1)*cos(t3)*sin(t2)*sin(t4)*sin(t5) + 0.00084023437500000005238864897449957*cos(t1)*cos(t4)*sin(t2)*sin(t3)*sin(t5)) + 0.5*(0.0016804687500000001047772979489991*cos(t2)*cos(t3)*sin(t1)*sin(t4)*sin(t5) + 0.0016804687500000001047772979489991*cos(t2)*cos(t4)*sin(t1)*sin(t3)*sin(t5) + 0.0016804687500000001047772979489991*cos(t3)*cos(t4)*sin(t1)*sin(t2)*sin(t5) - 0.0016804687500000001047772979489991*sin(t1)*sin(t2)*sin(t3)*sin(t4)*sin(t5))*(cos(t1)*cos(t5) - 1.0*cos(t2)*cos(t3)*cos(t4)*sin(t1)*sin(t5) + cos(t2)*sin(t1)*sin(t3)*sin(t4)*sin(t5) + cos(t3)*sin(t1)*sin(t2)*sin(t4)*sin(t5) + cos(t4)*sin(t1)*sin(t2)*sin(t3)*sin(t5)) + 0.5*(cos(t2)*cos(t3)*sin(t1)*sin(t4)*sin(t5) + cos(t2)*cos(t4)*sin(t1)*sin(t3)*sin(t5) + cos(t3)*cos(t4)*sin(t1)*sin(t2)*sin(t5) - 1.0*sin(t1)*sin(t2)*sin(t3)*sin(t4)*sin(t5))*(0.0016804687500000001047772979489991*cos(t1)*cos(t5) - 0.0016804687500000001047772979489991*cos(t2)*cos(t3)*cos(t4)*sin(t1)*sin(t5) + 0.0016804687500000001047772979489991*cos(t2)*sin(t1)*sin(t3)*sin(t4)*sin(t5) + 0.0016804687500000001047772979489991*cos(t3)*sin(t1)*sin(t2)*sin(t4)*sin(t5) + 0.0016804687500000001047772979489991*cos(t4)*sin(t1)*sin(t2)*sin(t3)*sin(t5))) + 1.0*td4*(0.5*(0.00084023437500000005238864897449957*cos(t1)*cos(t2)*cos(t3)*sin(t4)*sin(t5) + 0.00084023437500000005238864897449957*cos(t1)*cos(t2)*cos(t4)*sin(t3)*sin(t5) + 0.00084023437500000005238864897449957*cos(t1)*cos(t3)*cos(t4)*sin(t2)*sin(t5) - 0.00084023437500000005238864897449957*cos(t1)*sin(t2)*sin(t3)*sin(t4)*sin(t5))*(cos(t1)*cos(t2)*sin(t3)*sin(t4)*sin(t5) - 1.0*cos(t1)*cos(t2)*cos(t3)*cos(t4)*sin(t5) - 1.0*cos(t5)*sin(t1) + cos(t1)*cos(t3)*sin(t2)*sin(t4)*sin(t5) + cos(t1)*cos(t4)*sin(t2)*sin(t3)*sin(t5)) + 0.5*(cos(t1)*cos(t2)*cos(t3)*sin(t4)*sin(t5) + cos(t1)*cos(t2)*cos(t4)*sin(t3)*sin(t5) + cos(t1)*cos(t3)*cos(t4)*sin(t2)*sin(t5) - 1.0*cos(t1)*sin(t2)*sin(t3)*sin(t4)*sin(t5))*(0.00084023437500000005238864897449957*cos(t1)*cos(t2)*sin(t3)*sin(t4)*sin(t5) - 0.00084023437500000005238864897449957*cos(t1)*cos(t2)*cos(t3)*cos(t4)*sin(t5) - 0.00084023437500000005238864897449957*cos(t5)*sin(t1) + 0.00084023437500000005238864897449957*cos(t1)*cos(t3)*sin(t2)*sin(t4)*sin(t5) + 0.00084023437500000005238864897449957*cos(t1)*cos(t4)*sin(t2)*sin(t3)*sin(t5)) + 0.5*(0.0016804687500000001047772979489991*cos(t2)*cos(t3)*sin(t1)*sin(t4)*sin(t5) + 0.0016804687500000001047772979489991*cos(t2)*cos(t4)*sin(t1)*sin(t3)*sin(t5) + 0.0016804687500000001047772979489991*cos(t3)*cos(t4)*sin(t1)*sin(t2)*sin(t5) - 0.0016804687500000001047772979489991*sin(t1)*sin(t2)*sin(t3)*sin(t4)*sin(t5))*(cos(t1)*cos(t5) - 1.0*cos(t2)*cos(t3)*cos(t4)*sin(t1)*sin(t5) + cos(t2)*sin(t1)*sin(t3)*sin(t4)*sin(t5) + cos(t3)*sin(t1)*sin(t2)*sin(t4)*sin(t5) + cos(t4)*sin(t1)*sin(t2)*sin(t3)*sin(t5)) + 0.5*(cos(t2)*cos(t3)*sin(t1)*sin(t4)*sin(t5) + cos(t2)*cos(t4)*sin(t1)*sin(t3)*sin(t5) + cos(t3)*cos(t4)*sin(t1)*sin(t2)*sin(t5) - 1.0*sin(t1)*sin(t2)*sin(t3)*sin(t4)*sin(t5))*(0.0016804687500000001047772979489991*cos(t1)*cos(t5) - 0.0016804687500000001047772979489991*cos(t2)*cos(t3)*cos(t4)*sin(t1)*sin(t5) + 0.0016804687500000001047772979489991*cos(t2)*sin(t1)*sin(t3)*sin(t4)*sin(t5) + 0.0016804687500000001047772979489991*cos(t3)*sin(t1)*sin(t2)*sin(t4)*sin(t5) + 0.0016804687500000001047772979489991*cos(t4)*sin(t1)*sin(t2)*sin(t3)*sin(t5)))) + td5*(td6*(0.5*(0.0016804687500000001047772979489991*cos(t1)*cos(t5) - 0.0016804687500000001047772979489991*cos(t2)*cos(t3)*cos(t4)*sin(t1)*sin(t5) + 0.0016804687500000001047772979489991*cos(t2)*sin(t1)*sin(t3)*sin(t4)*sin(t5) + 0.0016804687500000001047772979489991*cos(t3)*sin(t1)*sin(t2)*sin(t4)*sin(t5) + 0.0016804687500000001047772979489991*cos(t4)*sin(t1)*sin(t2)*sin(t3)*sin(t5))*(cos(t2)*cos(t5)*sin(t1)*sin(t3)*sin(t4) - 1.0*cos(t2)*cos(t3)*cos(t4)*cos(t5)*sin(t1) - 1.0*cos(t1)*sin(t5) + cos(t3)*cos(t5)*sin(t1)*sin(t2)*sin(t4) + cos(t4)*cos(t5)*sin(t1)*sin(t2)*sin(t3)) + 0.5*(sin(t1)*sin(t5) - 1.0*cos(t1)*cos(t2)*cos(t3)*cos(t4)*cos(t5) + cos(t1)*cos(t2)*cos(t5)*sin(t3)*sin(t4) + cos(t1)*cos(t3)*cos(t5)*sin(t2)*sin(t4) + cos(t1)*cos(t4)*cos(t5)*sin(t2)*sin(t3))*(0.00084023437500000005238864897449957*cos(t1)*cos(t2)*sin(t3)*sin(t4)*sin(t5) - 0.00084023437500000005238864897449957*cos(t1)*cos(t2)*cos(t3)*cos(t4)*sin(t5) - 0.00084023437500000005238864897449957*cos(t5)*sin(t1) + 0.00084023437500000005238864897449957*cos(t1)*cos(t3)*sin(t2)*sin(t4)*sin(t5) + 0.00084023437500000005238864897449957*cos(t1)*cos(t4)*sin(t2)*sin(t3)*sin(t5)) + 0.5*(0.00084023437500000005238864897449957*sin(t1)*sin(t5) - 0.00084023437500000005238864897449957*cos(t1)*cos(t2)*cos(t3)*cos(t4)*cos(t5) + 0.00084023437500000005238864897449957*cos(t1)*cos(t2)*cos(t5)*sin(t3)*sin(t4) + 0.00084023437500000005238864897449957*cos(t1)*cos(t3)*cos(t5)*sin(t2)*sin(t4) + 0.00084023437500000005238864897449957*cos(t1)*cos(t4)*cos(t5)*sin(t2)*sin(t3))*(cos(t1)*cos(t2)*sin(t3)*sin(t4)*sin(t5) - 1.0*cos(t1)*cos(t2)*cos(t3)*cos(t4)*sin(t5) - 1.0*cos(t5)*sin(t1) + cos(t1)*cos(t3)*sin(t2)*sin(t4)*sin(t5) + cos(t1)*cos(t4)*sin(t2)*sin(t3)*sin(t5)) + 0.5*(0.0016804687500000001047772979489991*cos(t2)*cos(t5)*sin(t1)*sin(t3)*sin(t4) - 0.0016804687500000001047772979489991*cos(t2)*cos(t3)*cos(t4)*cos(t5)*sin(t1) - 0.0016804687500000001047772979489991*cos(t1)*sin(t5) + 0.0016804687500000001047772979489991*cos(t3)*cos(t5)*sin(t1)*sin(t2)*sin(t4) + 0.0016804687500000001047772979489991*cos(t4)*cos(t5)*sin(t1)*sin(t2)*sin(t3))*(cos(t1)*cos(t5) - 1.0*cos(t2)*cos(t3)*cos(t4)*sin(t1)*sin(t5) + cos(t2)*sin(t1)*sin(t3)*sin(t4)*sin(t5) + cos(t3)*sin(t1)*sin(t2)*sin(t4)*sin(t5) + cos(t4)*sin(t1)*sin(t2)*sin(t3)*sin(t5))) + 1.0*td1*(0.00021005859375000001309716224362489*cos(2.0*t2)*cos(2.0*t3)*sin(2.0*t1)*sin(2.0*t4)*sin(t5) + 0.00021005859375000001309716224362489*cos(2.0*t2)*cos(2.0*t4)*sin(2.0*t1)*sin(2.0*t3)*sin(t5) + 0.00021005859375000001309716224362489*cos(2.0*t3)*cos(2.0*t4)*sin(2.0*t1)*sin(2.0*t2)*sin(t5) - 0.00042011718750000002619432448724979*cos(2.0*t1)*cos(t2)*cos(t3)*cos(t5)*sin(t4) - 0.00042011718750000002619432448724979*cos(2.0*t1)*cos(t2)*cos(t4)*cos(t5)*sin(t3) - 0.00042011718750000002619432448724979*cos(2.0*t1)*cos(t3)*cos(t4)*cos(t5)*sin(t2) - 0.00021005859375000001309716224362489*sin(2.0*t1)*sin(2.0*t2)*sin(2.0*t3)*sin(2.0*t4)*sin(t5) + 0.00042011718750000002619432448724979*cos(2.0*t1)*cos(t5)*sin(t2)*sin(t3)*sin(t4)) + td2*(0.00063017578125000003929148673087468*cos(2.0*t2)*cos(2.0*t3)*cos(2.0*t4)*sin(t5) - 0.00042011718750000002619432448724979*cos(t1)^2*sin(t5) - 0.00042011718750000002619432448724979*sin(t5) - 0.00063017578125000003929148673087468*cos(2.0*t2)*sin(2.0*t3)*sin(2.0*t4)*sin(t5) - 0.00063017578125000003929148673087468*cos(2.0*t3)*sin(2.0*t2)*sin(2.0*t4)*sin(t5) - 0.00063017578125000003929148673087468*cos(2.0*t4)*sin(2.0*t2)*sin(2.0*t3)*sin(t5) - 0.00021005859375000001309716224362489*cos(2.0*t1)*cos(2.0*t2)*cos(2.0*t3)*cos(2.0*t4)*sin(t5) + 0.00021005859375000001309716224362489*cos(2.0*t1)*cos(2.0*t2)*sin(2.0*t3)*sin(2.0*t4)*sin(t5) + 0.00021005859375000001309716224362489*cos(2.0*t1)*cos(2.0*t3)*sin(2.0*t2)*sin(2.0*t4)*sin(t5) + 0.00021005859375000001309716224362489*cos(2.0*t1)*cos(2.0*t4)*sin(2.0*t2)*sin(2.0*t3)*sin(t5) - 0.00021005859375000001309716224362489*sin(2.0*t1)*cos(t2)*cos(t3)*cos(t4)*cos(t5) + 0.00021005859375000001309716224362489*sin(2.0*t1)*cos(t2)*cos(t5)*sin(t3)*sin(t4) + 0.00021005859375000001309716224362489*sin(2.0*t1)*cos(t3)*cos(t5)*sin(t2)*sin(t4) + 0.00021005859375000001309716224362489*sin(2.0*t1)*cos(t4)*cos(t5)*sin(t2)*sin(t3) - 0.00042011718750000002619432448724979*cos(t1)*cos(t2)*cos(t3)*cos(t4)*cos(t5)*sin(t1) + 0.00042011718750000002619432448724979*cos(t1)*cos(t2)*cos(t5)*sin(t1)*sin(t3)*sin(t4) + 0.00042011718750000002619432448724979*cos(t1)*cos(t3)*cos(t5)*sin(t1)*sin(t2)*sin(t4) + 0.00042011718750000002619432448724979*cos(t1)*cos(t4)*cos(t5)*sin(t1)*sin(t2)*sin(t3)) + td3*(0.00063017578125000003929148673087468*cos(2.0*t2)*cos(2.0*t3)*cos(2.0*t4)*sin(t5) - 0.00042011718750000002619432448724979*cos(t1)^2*sin(t5) - 0.00042011718750000002619432448724979*sin(t5) - 0.00063017578125000003929148673087468*cos(2.0*t2)*sin(2.0*t3)*sin(2.0*t4)*sin(t5) - 0.00063017578125000003929148673087468*cos(2.0*t3)*sin(2.0*t2)*sin(2.0*t4)*sin(t5) - 0.00063017578125000003929148673087468*cos(2.0*t4)*sin(2.0*t2)*sin(2.0*t3)*sin(t5) - 0.00021005859375000001309716224362489*cos(2.0*t1)*cos(2.0*t2)*cos(2.0*t3)*cos(2.0*t4)*sin(t5) + 0.00021005859375000001309716224362489*cos(2.0*t1)*cos(2.0*t2)*sin(2.0*t3)*sin(2.0*t4)*sin(t5) + 0.00021005859375000001309716224362489*cos(2.0*t1)*cos(2.0*t3)*sin(2.0*t2)*sin(2.0*t4)*sin(t5) + 0.00021005859375000001309716224362489*cos(2.0*t1)*cos(2.0*t4)*sin(2.0*t2)*sin(2.0*t3)*sin(t5) - 0.00021005859375000001309716224362489*sin(2.0*t1)*cos(t2)*cos(t3)*cos(t4)*cos(t5) + 0.00021005859375000001309716224362489*sin(2.0*t1)*cos(t2)*cos(t5)*sin(t3)*sin(t4) + 0.00021005859375000001309716224362489*sin(2.0*t1)*cos(t3)*cos(t5)*sin(t2)*sin(t4) + 0.00021005859375000001309716224362489*sin(2.0*t1)*cos(t4)*cos(t5)*sin(t2)*sin(t3) - 0.00042011718750000002619432448724979*cos(t1)*cos(t2)*cos(t3)*cos(t4)*cos(t5)*sin(t1) + 0.00042011718750000002619432448724979*cos(t1)*cos(t2)*cos(t5)*sin(t1)*sin(t3)*sin(t4) + 0.00042011718750000002619432448724979*cos(t1)*cos(t3)*cos(t5)*sin(t1)*sin(t2)*sin(t4) + 0.00042011718750000002619432448724979*cos(t1)*cos(t4)*cos(t5)*sin(t1)*sin(t2)*sin(t3)) + td4*(0.00063017578125000003929148673087468*cos(2.0*t2)*cos(2.0*t3)*cos(2.0*t4)*sin(t5) - 0.00042011718750000002619432448724979*cos(t1)^2*sin(t5) - 0.00042011718750000002619432448724979*sin(t5) - 0.00063017578125000003929148673087468*cos(2.0*t2)*sin(2.0*t3)*sin(2.0*t4)*sin(t5) - 0.00063017578125000003929148673087468*cos(2.0*t3)*sin(2.0*t2)*sin(2.0*t4)*sin(t5) - 0.00063017578125000003929148673087468*cos(2.0*t4)*sin(2.0*t2)*sin(2.0*t3)*sin(t5) - 0.00021005859375000001309716224362489*cos(2.0*t1)*cos(2.0*t2)*cos(2.0*t3)*cos(2.0*t4)*sin(t5) + 0.00021005859375000001309716224362489*cos(2.0*t1)*cos(2.0*t2)*sin(2.0*t3)*sin(2.0*t4)*sin(t5) + 0.00021005859375000001309716224362489*cos(2.0*t1)*cos(2.0*t3)*sin(2.0*t2)*sin(2.0*t4)*sin(t5) + 0.00021005859375000001309716224362489*cos(2.0*t1)*cos(2.0*t4)*sin(2.0*t2)*sin(2.0*t3)*sin(t5) - 0.00021005859375000001309716224362489*sin(2.0*t1)*cos(t2)*cos(t3)*cos(t4)*cos(t5) + 0.00021005859375000001309716224362489*sin(2.0*t1)*cos(t2)*cos(t5)*sin(t3)*sin(t4) + 0.00021005859375000001309716224362489*sin(2.0*t1)*cos(t3)*cos(t5)*sin(t2)*sin(t4) + 0.00021005859375000001309716224362489*sin(2.0*t1)*cos(t4)*cos(t5)*sin(t2)*sin(t3) - 0.00042011718750000002619432448724979*cos(t1)*cos(t2)*cos(t3)*cos(t4)*cos(t5)*sin(t1) + 0.00042011718750000002619432448724979*cos(t1)*cos(t2)*cos(t5)*sin(t1)*sin(t3)*sin(t4) + 0.00042011718750000002619432448724979*cos(t1)*cos(t3)*cos(t5)*sin(t1)*sin(t2)*sin(t4) + 0.00042011718750000002619432448724979*cos(t1)*cos(t4)*cos(t5)*sin(t1)*sin(t2)*sin(t3)))];
